simulink model "fxpdemo_prelookup_interpolation"  (Simulink 7.6)
settings: Solver=FixedStepDiscrete  StartTime=0.0  StopTime=10.0  RelTol=1e-3
libraries: simulink x2
Description:
  | Fixed-Point Prelookup and Interpolation
  | 
  | * Prelookup and Interpolation Using Prelookup blocks support both floating-point data
  | types and fixed-point data types.
  | * The algorithms that perform fraction calculation and evenly-spaced index search do not saturate.
  | Therefore, the Prelookup block does not have a saturation parameter. Press *Ctrl+b* to
  | generate code for the demo model. Observe the saturation-free algorithms in the generated code.
  | * Even if the *Saturate on integer overflow* parameter is checked, the algorithms that perform
  | interpolation will saturate only when the *Intermediate results data type* cannot hold the intermediate
  | results, or the *Output data type* can not hold the result. Press *Ctrl+b* to generate code for the demo
  | model. Observe the saturation-free algorithms in the generated code.
  | * Prelookup and Interpolation Using Prelookup blocks support all rounding modes, including |Simplest|
  | rounding mode. Double-click the blocks to open their dialogs and specify the rounding modes.
  | * When evenly-spaced index search is used with breakpoints spaced apart by a power of two in Prelookup
  | blocks, the division needed to calculate indices is optimized using an efficient shift operation in
  | the generated code.
  | * Simulink(R) always checks dimensional consistency between the *Breakpoint data* parameter of the Prelookup
  | block and the *Table data* parameter of the Interpolation Using Prelookup block.
  | * Prelookup and Interpolation Using Prelookup blocks support two different indexing conventions,
  | specified by the *Use last breakpoint for input at or above upper limit* parameter in the Prelookup
  | block and the *Valid index input may reach last index* parameter in the Interpolation Using Prelookup
  | block. Simulink(R) always checks the consistency of indexing conventions between these blocks.
settings Model: Creator=The MathWorks Inc.  ExtModeAutoUpdateStatusClock=off
settings DataIOCC: SaveFormat=StructureWithTime
settings OptimizationCC: InlineParams=on  InlineInvariantSignals=on  InitFltsAndDblsToZero=on  OptimizeModelRefInitCode=on  LifeSpan=1
settings DebuggingCC: SaveWithParameterizedLinksMsg=none  SignalResolutionControl=TryResolveAllWithWarning  ParameterDowncastMsg=none  ParameterOverflowMsg=none  ParameterPrecisionLossMsg=none  StrictBusMsg=Warning
settings HardwareCC: TargetEndianess=LittleEndian  TargetHWDeviceType=Generic->MATLAB Host Computer  ProdEqTarget=off
settings RTWCC: SystemTargetFile=ert.tlc  TemplateMakefile=ert_default_tmf  Description=Real-Time Workshop Embedded Coder (no auto configuration)  GenerateReport=on  ProcessScript=ert_make_rtw_hook  IncludeHyperlinkInReport=on  LaunchReport=on  IncludeERTFirstTime=on
settings CodeAppCC: IgnoreCustomStorageClasses=off
settings ERTTargetCC: TargetFcnLib=ansi_tfl_tmw.mat  MultiwordLength=2048  GenerateSampleERTMain=on  MatFileLogging=on  InlinedParameterPlacement=NonHierarchical  ERTCustomFileTemplate=example_file_process.tlc  ConvertIfToSwitch=off

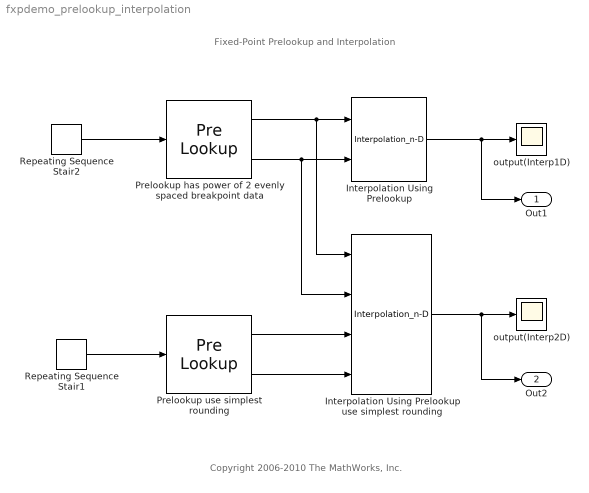
== system fxpdemo_prelookup_interpolation ==
  note: Copyright 2006-2010 The MathWorks, Inc.
  note: Fixed-Point Prelookup and Interpolation
  Interpolation Using Prelookup : Interpolation_n-D  NumberOfTableDimensions=1  Table=reshape([1:11], 1,11)  ExtrapMethod=None - Clip  ValidIndexMayReachLast=on  OutDataTypeStr=fixdt(1, 16, 1.*2^-3, 5)  SaturateOnIntegerOverflow=on
      settings: InputPortMap=u0,u1
  Interpolation Using Prelookup use simplest rounding : Interpolation_n-D  ExtrapMethod=None - Clip  ValidIndexMayReachLast=on  OutDataTypeStr=fixdt(1,16,5)  RndMeth=Simplest  SaturateOnIntegerOverflow=on
  Prelookup has power of 2 evenly spaced breakpoint data : PreLookup  BreakpointsData=[1:11]  IndexSearchMethod=Evenly spaced points  BeginIndexSearchUsingPreviousIndexResult=on  UseLastBreakpoint=on
  Prelookup use simplest rounding : PreLookup  BreakpointsData=[1:11]  IndexSearchMethod=Linear search  BeginIndexSearchUsingPreviousIndexResult=on  UseLastBreakpoint=on  IndexDataTypeStr=uint8  FractionDataTypeStr=fixdt(0,16,14)  RndMeth=Simplest
  Repeating Sequence Stair1 : simulink/Sources/Repeating Sequence Stair  SystemSampleTime=-1  OutValues=[-1:0.1:11]  tsamp=0.01  OutMin=[]  OutMax=[]  OutDataTypeStr=fixdt(1,16,5)  OutputDataTypeScalingMode=Specify via dialog  OutDataType=sfix(16)  ConRadixGroup=Use specified scaling  OutScaling=2^-5
  Repeating Sequence Stair2 : simulink/Sources/Repeating Sequence Stair  SystemSampleTime=-1  OutValues=[-1:0.1:11]  tsamp=0.01  OutMin=[]  OutMax=[]  OutDataTypeStr=fixdt(1,32,24)  OutputDataTypeScalingMode=Specify via dialog  OutDataType=sfix(32)  ConRadixGroup=Use specified scaling  OutScaling=2^-24
  output(Interp1D) : Scope
      settings: TimeRange=10  YMin=0  YMax=12
  output(Interp2D) : Scope
      settings: TimeRange=10  YMin=0  YMax=12
  Out1 : Outport
  Out2 : Outport  Port=2
  wires:
  Repeating Sequence Stair2/1 -> Prelookup has power of 2 evenly spaced breakpoint data/1
  Prelookup has power of 2 evenly spaced breakpoint data/1 -> Interpolation Using Prelookup/1, Interpolation Using Prelookup use simplest rounding/1
  Prelookup has power of 2 evenly spaced breakpoint data/2 -> Interpolation Using Prelookup/2, Interpolation Using Prelookup use simplest rounding/2
  Interpolation Using Prelookup/1 -> output(Interp1D)/1, Out1/1
  Interpolation Using Prelookup use simplest rounding/1 -> output(Interp2D)/1, Out2/1
  Repeating Sequence Stair1/1 -> Prelookup use simplest rounding/1
  Prelookup use simplest rounding/1 -> Interpolation Using Prelookup use simplest rounding/3
  Prelookup use simplest rounding/2 -> Interpolation Using Prelookup use simplest rounding/4
